simulink model "modulationsarten"  (Simulink 8.1)
settings: Solver=VariableStepDiscrete  StartTime=0.0  StopTime=simulationTime  RelTol=1e-3
values from neighbouring files (symbols this model uses):
  lengthOfSymbol = 64    [GSM_sim_ISI_config.m]    (also in GSM_sim_config.m; modulationsarten_config.m)
  sampleTime = 1    [GSM_sim_ISI_config.m]    (also in GSM_sim_config.m; modulationsarten_config.m)
libraries: commchan3 x4, commdigbbndpm3 x2, commdigbbndcpm2 x2, commfilt2 x2, commutil2 x1, dspsigops x1
settings Model: Creator=Philipp Fetzer  LastModifiedBy=mainster
settings DebuggingCC: SolverPrmCheckMsg=none  StrictBusMsg=Warning

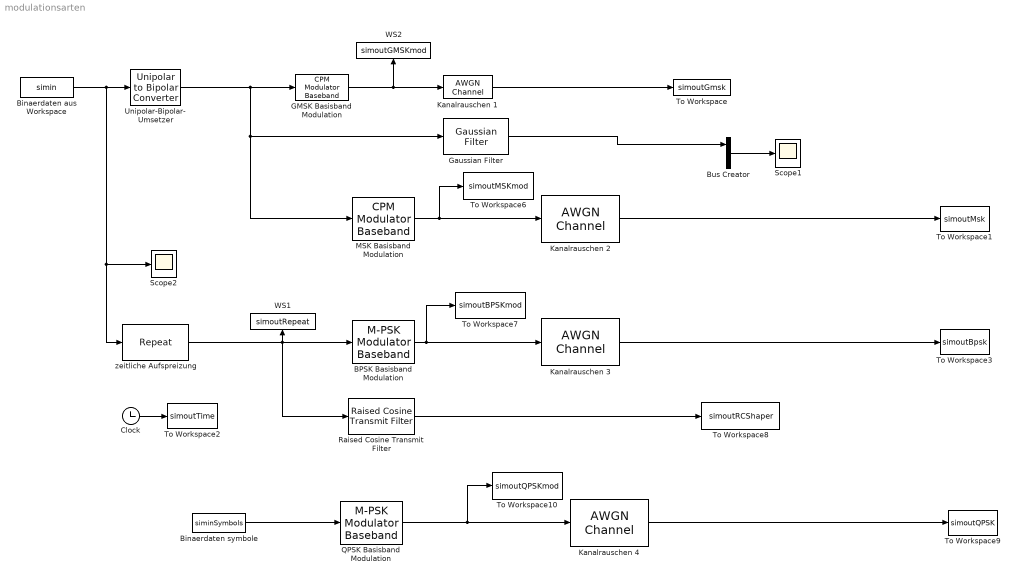
== system modulationsarten ==
  BPSK Basisband Modulation : commdigbbndpm3/M-PSK Modulator Baseband  M=2  InType=Integer  Enc=Binary  Mapping=[0:2]  Ph=phaseOffset  outDtype=double  outWordLen=16  outUDDataType=sfix(16)  outFracLenMode=Best precision  outFracLen=15
  Binaerdaten aus Workspace : FromWorkspace  VariableName=simin  SampleTime=sampleTime
  Binaerdaten symbole : FromWorkspace  VariableName=siminSymbols  SampleTime=sampleTime
  Bus Creator : BusCreator  Inputs=2
  Clock : Clock
  GMSK Basisband Modulation : commdigbbndcpm2/CPM Modulator Baseband  Mnum=2  inputType=Integer  mappingType=Binary  modIdx=.5  pulseShape=Gaussian  BT=.3  mainLobePulseLength=0.2  rollOff=0.2  pulseLength=4  preHistory=1  phaseOffset=phaseOffset  samplesPerSymbol=lengthOfSymbol  RateOptions=Inherit from input (this choice will be removed - see release notes)  outDataType=double
  Gaussian Filter : commfilt2/Gaussian Filter  N=lengthOfSymbol  BT=0.3  D=2  sampMode=Frame-based  normMode=Filter energy  filterGain=1  checkCoeff=off  variableName=gaussFilt  launchFVT=off  roundingMode=Floor  overflowMode=off  InputProcessing=Columns as channels (frame based)
  Kanalrauschen {1..4} (4 alike) : commchan3/AWGN Channel  InputProcessing=Inherited (this choice will be removed - see release notes)  seed=67  noiseMode="Signal to noise ratio  (SNR)"  EbNodB=30  EsNodB=10  SNRdB=SNR  bitsPerSym=1  Ps=1  Tsym=1  variance=1
  MSK Basisband Modulation : commdigbbndcpm2/CPM Modulator Baseband  Mnum=2  inputType=Integer  mappingType=Binary  modIdx=0.5  pulseShape=Rectangular  BT=0.3  mainLobePulseLength=0.2  rollOff=0.2  pulseLength=1  preHistory=1  phaseOffset=phaseOffset  samplesPerSymbol=lengthOfSymbol  RateOptions=Inherit from input (this choice will be removed - see release notes)  outDataType=double
  QPSK Basisband Modulation : commdigbbndpm3/M-PSK Modulator Baseband  M=4  InType=Integer  Enc=Binary  Mapping=[0:2]  Ph=phaseOffset  outDtype=double  outWordLen=16  outUDDataType=sfix(16)  outFracLenMode=Best precision  outFracLen=15
  Raised Cosine Transmit Filter : commfilt2/Raised Cosine Transmit Filter  filtType=Normal  D=5  R=0.8  sampMode=Mute  saveAsFlag=0  N=64  framing=Enforce single-rate processing  InputProcessing=Columns as channels (frame based)  checkGain=Normalized  filterGain=1  checkCoeff=off  variableName=rcTxFilt  launchFVT=off  roundingMode=Floor  overflowMode=off
  Scope1 : Scope
      settings: ShowLegends=on  TimeRange=150  YMin=-2  YMax=3
  Scope2 : Scope
      settings: SaveName=ScopeData2
  To Workspace : ToWorkspace  VariableName=simoutGmsk  SampleTime=-1  SaveFormat=Structure
  To Workspace1 : ToWorkspace  VariableName=simoutMsk  SampleTime=-1  SaveFormat=Structure
  To Workspace10 : ToWorkspace  VariableName=simoutQPSKmod  SampleTime=-1  SaveFormat=Structure
  To Workspace2 : ToWorkspace  VariableName=simoutTime  SampleTime=-1  SaveFormat=Structure
  To Workspace3 : ToWorkspace  VariableName=simoutBpsk  SampleTime=-1  SaveFormat=Structure
  To Workspace6 : ToWorkspace  VariableName=simoutMSKmod  SampleTime=-1  SaveFormat=Structure
  To Workspace7 : ToWorkspace  VariableName=simoutBPSKmod  SampleTime=-1  SaveFormat=Structure
  To Workspace8 : ToWorkspace  VariableName=simoutRCShaper  SampleTime=-1  SaveFormat=Structure
  To Workspace9 : ToWorkspace  VariableName=simoutQPSK  SampleTime=-1  SaveFormat=Structure
  Unipolar-Bipolar- Umsetzer : commutil2/Unipolar to Bipolar Converter  M=2  polarity=Positive  dataType=Inherit via internal rule
  WS1 : ToWorkspace  VariableName=simoutRepeat  SampleTime=-1  SaveFormat=Structure
  WS2 : ToWorkspace  VariableName=simoutGMSKmod  SampleTime=-1  SaveFormat=Structure
  zeitliche Aufspreizung : dspsigops/Repeat  N=lengthOfSymbol  InputProcessing=Inherited (this choice will be removed - see release notes)  RateOptions=Allow multirate processing  ic=0  mode=Unused parameter value
  wires:
  Unipolar-Bipolar- Umsetzer/1 -> GMSK Basisband Modulation/1, MSK Basisband Modulation/1, Gaussian Filter/1
  MSK Basisband Modulation/1 -> Kanalrauschen 2/1, To Workspace6/1
  Binaerdaten aus Workspace/1 -> Unipolar-Bipolar- Umsetzer/1, Scope2/1, zeitliche Aufspreizung/1
  Clock/1 -> To Workspace2/1
  Kanalrauschen 1/1 -> To Workspace/1
  GMSK Basisband Modulation/1 -> WS2/1, Kanalrauschen 1/1
  BPSK Basisband Modulation/1 -> Kanalrauschen 3/1, To Workspace7/1
  Kanalrauschen 2/1 -> To Workspace1/1
  Kanalrauschen 3/1 -> To Workspace3/1
  zeitliche Aufspreizung/1 -> BPSK Basisband Modulation/1, Raised Cosine Transmit Filter/1, WS1/1
  Raised Cosine Transmit Filter/1 -> To Workspace8/1
  QPSK Basisband Modulation/1 -> Kanalrauschen 4/1, To Workspace10/1
  Kanalrauschen 4/1 -> To Workspace9/1
  Binaerdaten symbole/1 -> QPSK Basisband Modulation/1
  Bus Creator/1 -> Scope1/1
  Gaussian Filter/1 -> Bus Creator/1
